simulink model "Copy_of_exercise_4_openLoop"  (R2018a)
settings: Solver=VariableStepAuto  StartTime=0.0  StopTime=0.01  RelTol=1e-3
undefined symbols (not defined in the file or in its folder): p
settings Model: Creator=mz-171742  LastModifiedBy=mz-171742

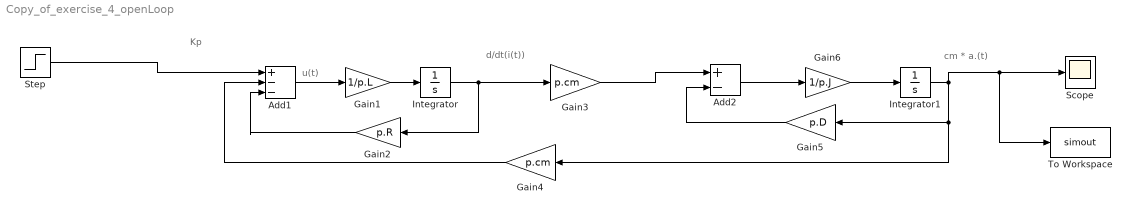
== system Copy_of_exercise_4_openLoop ==
  note: d/dt(i(t))
  note: cm * a.(t)
  note: u(t)
  note: Kp
  Add1 : Sum  Inputs=+--
  Add2 : Sum  Inputs=+-
  Gain1 : Gain  Gain=1/p.L
  Gain2 : Gain  Gain=p.R
  Gain3 : Gain  Gain=p.cm
  Gain4 : Gain  Gain=p.cm
  Gain5 : Gain  Gain=p.D
  Gain6 : Gain  Gain=1/p.J
  Integrator : Integrator
  Integrator1 : Integrator
  Scope : Scope
  Step : Step  Time=0  SampleTime=0
  To Workspace : ToWorkspace  VariableName=simout  SaveFormat=Structure With Time  SampleTime=-1
  wires:
  Integrator/1 -> Gain2/1, Gain3/1
  Add1/1 -> Gain1/1
  Integrator1/1 -> To Workspace/1, Scope/1, Gain4/1, Gain5/1
  Gain1/1 -> Integrator/1
  Gain2/1 -> Add1/3
  Gain3/1 -> Add2/1
  Add2/1 -> Gain6/1
  Gain4/1 -> Add1/2
  Gain5/1 -> Add2/2
  Gain6/1 -> Integrator1/1
  Step/1 -> Add1/1
